simulink model "case14"  (R2018b)
settings: Solver=VariableStepAuto  StartTime=0.0  StopTime=10.0  RelTol=1e-3
(part 1 of 2)
settings Model: Creator=yogita.g  LastModifiedBy=nishanthkumar.l
settings DataIOCC: SaveCompleteFinalSimState=on

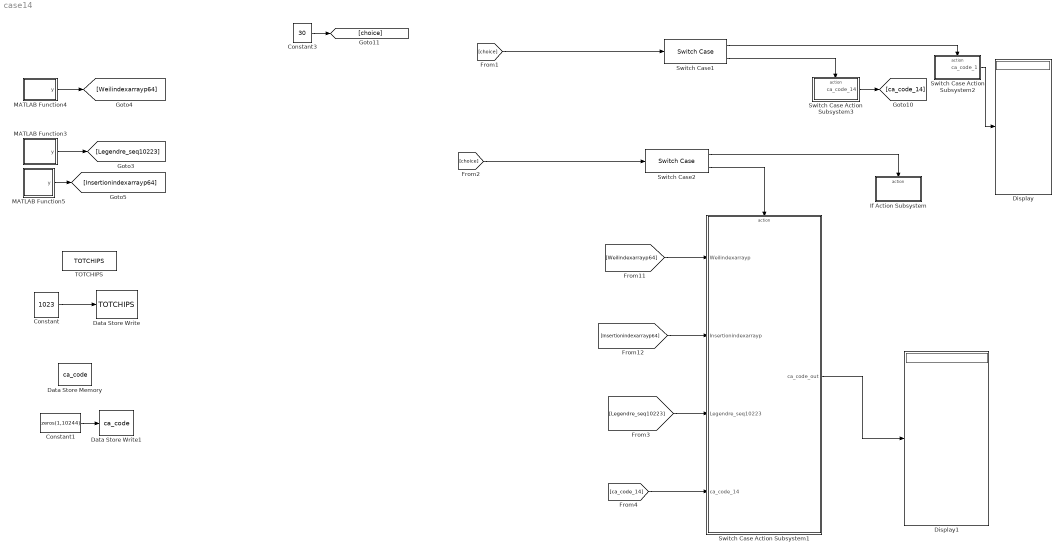
== system case14 ==
  Constant : Constant  Value=1023  VectorParams1D=off  OutDataTypeStr=int32  SampleTime=-1
  Constant1 : Constant  Value=zeros(1,10244)
  Constant3 : Constant  Value=30
  Data Store Memory : DataStoreMemory  DataStoreName=ca_code  ReadBeforeWriteMsg=warning  WriteAfterWriteMsg=warning  WriteAfterReadMsg=warning  ShowAdditionalParam=off  Dimensions=[1 10244]
  Data Store Write : DataStoreWrite  DataStoreName=TOTCHIPS
  Data Store Write1 : DataStoreWrite  DataStoreName=ca_code
  Display : Display
  Display1 : Display
  If Action Subsystem : Subsystem  TreatAsAtomicUnit=on
  MATLAB Function3 : MATLAB Function  TreatAsAtomicUnit=on
  MATLAB Function4 : MATLAB Function  TreatAsAtomicUnit=on
  MATLAB Function5 : MATLAB Function  TreatAsAtomicUnit=on
  Switch Case Action Subsystem1 : Subsystem  TreatAsAtomicUnit=on
  Switch Case Action Subsystem2 : Subsystem  TreatAsAtomicUnit=on
  Switch Case Action Subsystem3 : Subsystem  TreatAsAtomicUnit=on
  Switch Case1 : SwitchCase  CaseConditions={1,14}  ShowDefaultCase=off
  Switch Case2 : SwitchCase  CaseConditions={1,14}  ShowDefaultCase=off
  TOTCHIPS : DataStoreMemory  DataStoreName=TOTCHIPS  ReadBeforeWriteMsg=warning  WriteAfterWriteMsg=warning  WriteAfterReadMsg=warning  ShowAdditionalParam=off  OutDataTypeStr=int32
  wires:
  MATLAB Function5/1(y) -> [Insertionindexarrayp64]
  MATLAB Function4/1(y) -> [Weilindexarrayp64]
  MATLAB Function3/1(y) -> [Legendre_seq10223]
  Switch Case1/1 -> Switch Case Action Subsystem2/Action
  Switch Case1/2 -> Switch Case Action Subsystem3/Action
  Switch Case Action Subsystem3/1(ca_code_14) -> [ca_code_14]
  [choice] -> Switch Case1/1
  Constant3/1 -> [choice]
  Constant/1 -> Data Store Write/1
  Switch Case Action Subsystem2/1(ca_code_1) -> Display/1
  [Weilindexarrayp64] -> Switch Case Action Subsystem1/1(Weilindexarrayp)
  [ca_code_14] -> Switch Case Action Subsystem1/4(ca_code_14)
  [Legendre_seq10223] -> Switch Case Action Subsystem1/3(Legendre_seq10223)
  [Insertionindexarrayp64] -> Switch Case Action Subsystem1/2(Insertionindexarrayp)
  [choice] -> Switch Case2/1
  Switch Case2/2 -> Switch Case Action Subsystem1/Action
  Switch Case2/1 -> If Action Subsystem/Action
  Switch Case Action Subsystem1/1(ca_code_out) -> Display1/1
  Constant1/1 -> Data Store Write1/1

== system case14/If Action Subsystem ==
  Action Port : ActionPort  ActionType=case

== system case14/Switch Case Action Subsystem1 ==
  Weilindexarrayp : Inport
  Insertionindexarrayp : Inport  Port=2
  Legendre_seq10223 : Inport  Port=3
  ca_code_14 : Inport  Port=4
  Action Port : ActionPort  ActionType=case
  For Iterator Subsystem : Subsystem  TreatAsAtomicUnit=on
  ca_code_out : Outport
  wires:
  Weilindexarrayp/1 -> For Iterator Subsystem/1(Weilindexarrayp)
  Insertionindexarrayp/1 -> For Iterator Subsystem/2(Insertionindexarrayp)
  For Iterator Subsystem/1(ca_code) -> ca_code_out/1
  Legendre_seq10223/1 -> For Iterator Subsystem/3(Legendre_seq10223)
  ca_code_14/1 -> For Iterator Subsystem/4(ca_code_14)

== system case14/Switch Case Action Subsystem2 ==
  Action Port : ActionPort  ActionType=case
  MATLAB Function : MATLAB Function  TreatAsAtomicUnit=on
  ca_code_1 : Outport
  wires:
  MATLAB Function/1(ca_code) -> ca_code_1/1

== system case14/Switch Case Action Subsystem3 ==
  Action Port : ActionPort  ActionType=case
  MATLAB Function : MATLAB Function  TreatAsAtomicUnit=on
  ca_code_14 : Outport
  wires:
  MATLAB Function/1(ca_code) -> ca_code_14/1

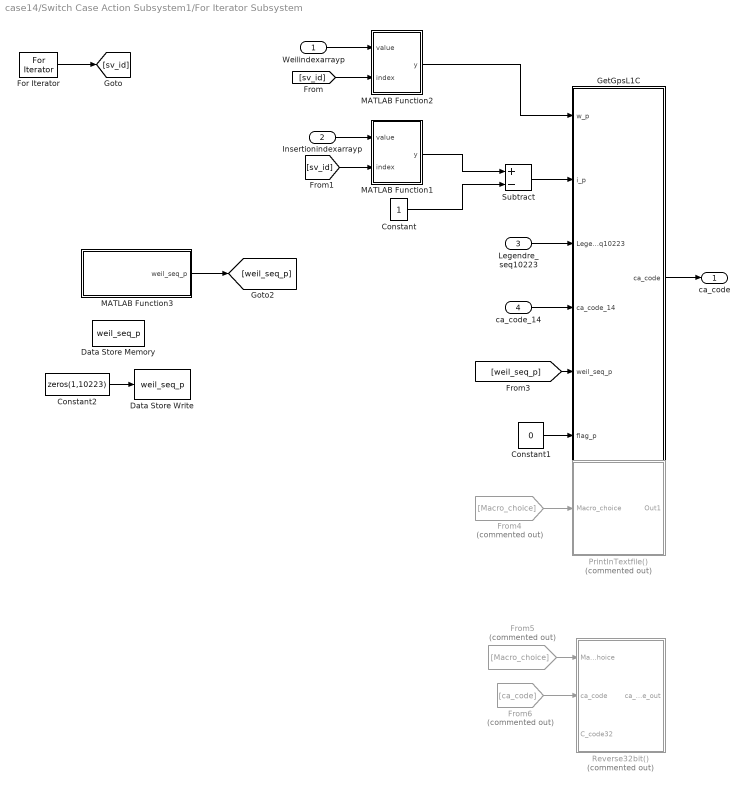
== system case14/Switch Case Action Subsystem1/For Iterator Subsystem ==
  Weilindexarrayp : Inport
  Insertionindexarrayp : Inport  Port=2  OutDataTypeStr=int32
  Legendre_seq10223 : Inport  Port=3
  ca_code_14 : Inport  Port=4
  Constant : Constant  VectorParams1D=off  OutDataTypeStr=int32  SampleTime=-1
  Constant1 : Constant  Value=0  OutDataTypeStr=int32
  Constant2 : Constant  Value=zeros(1,10223)
  Data Store Memory : DataStoreMemory  DataStoreName=weil_seq_p  ReadBeforeWriteMsg=warning  WriteAfterWriteMsg=warning  WriteAfterReadMsg=warning  ShowAdditionalParam=off  Dimensions=[1 10223]
  Data Store Write : DataStoreWrite  DataStoreName=weil_seq_p
  For Iterator : ForIterator  IterationLimit=1
  From4 : From  Commented=on  GotoTag=Macro_choice
  From5 : From  Commented=on  GotoTag=Macro_choice
  From6 : From  Commented=on  GotoTag=ca_code
  GetGpsL1C : Subsystem
  MATLAB Function1 : MATLAB Function  TreatAsAtomicUnit=on
  MATLAB Function2 : MATLAB Function  TreatAsAtomicUnit=on
  MATLAB Function3 : MATLAB Function  TreatAsAtomicUnit=on
  PrintInTextfile() : Subsystem  Commented=on
  Reverse32bit() : Subsystem  Commented=on
  Subtract : Sum  Inputs=+-
  ca_code : Outport
  wires:
  For Iterator/1 -> [sv_id]
  Weilindexarrayp/1 -> MATLAB Function2/1(value)
  [sv_id] -> MATLAB Function2/2(index)
  MATLAB Function2/1(y) -> GetGpsL1C/1(w_p)
  [sv_id] -> MATLAB Function1/2(index)
  Insertionindexarrayp/1 -> MATLAB Function1/1(value)
  From6/1 -> Reverse32bit()/2(ca_code)
  From5/1 -> Reverse32bit()/1(Macro_choice)
  From4/1 -> PrintInTextfile()/1(Macro_choice)
  Legendre_seq10223/1 -> GetGpsL1C/3(Legendre_seq10223)
  GetGpsL1C/1(ca_code) -> ca_code/1
  ca_code_14/1 -> GetGpsL1C/4(ca_code_14)
  [weil_seq_p] -> GetGpsL1C/5(weil_seq_p)
  MATLAB Function1/1(y) -> Subtract/1
  Constant/1 -> Subtract/2
  Subtract/1 -> GetGpsL1C/2(i_p)
  MATLAB Function3/1(weil_seq_p) -> [weil_seq_p]
  Constant1/1 -> GetGpsL1C/6(flag_p)
  Constant2/1 -> Data Store Write/1

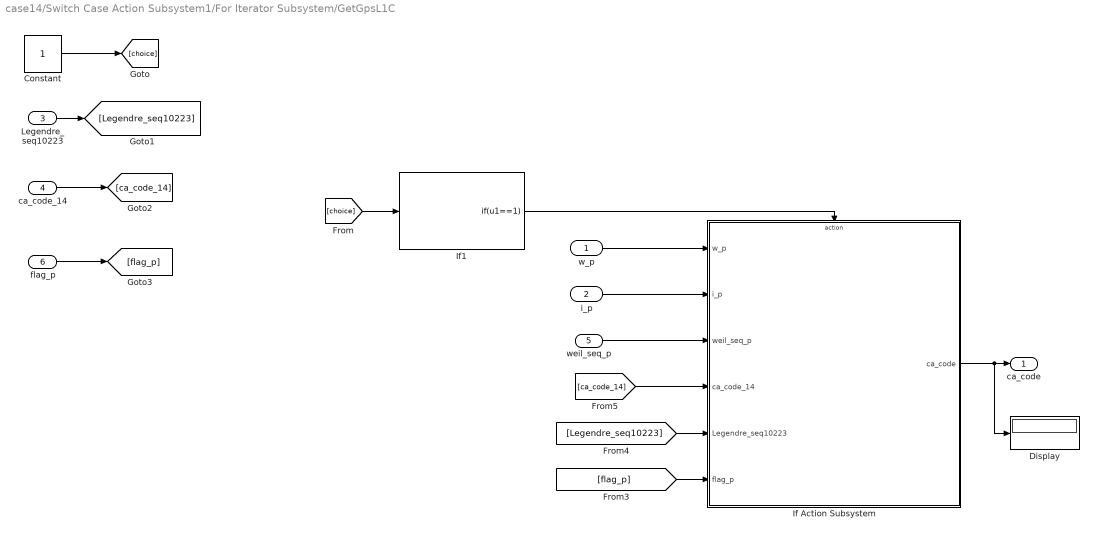
== system case14/Switch Case Action Subsystem1/For Iterator Subsystem/GetGpsL1C ==
  w_p : Inport
  i_p : Inport  Port=2
  Legendre_seq10223 : Inport  Port=3
  ca_code_14 : Inport  Port=4
  weil_seq_p : Inport  Port=5
  flag_p : Inport  Port=6  OutDataTypeStr=int32
  Constant : Constant  VectorParams1D=off  SampleTime=-1
  Display : Display
  If Action Subsystem : Subsystem  TreatAsAtomicUnit=on
  If1 : If  IfExpression=u1==1  ShowElse=off
  ca_code : Outport
  wires:
  If1/1 -> If Action Subsystem/Action
  i_p/1 -> If Action Subsystem/2(i_p)
  [Legendre_seq10223] -> If Action Subsystem/5(Legendre_seq10223)
  w_p/1 -> If Action Subsystem/1(w_p)
  [choice] -> If1/1
  Constant/1 -> [choice]
  Legendre_seq10223/1 -> [Legendre_seq10223]
  If Action Subsystem/1(ca_code) -> Display/1, ca_code/1
  ca_code_14/1 -> [ca_code_14]
  [ca_code_14] -> If Action Subsystem/4(ca_code_14)
  weil_seq_p/1 -> If Action Subsystem/3(weil_seq_p)
  flag_p/1 -> [flag_p]
  [flag_p] -> If Action Subsystem/6(flag_p)

== system case14/Switch Case Action Subsystem1/For Iterator Subsystem/PrintInTextfile() ==
  Macro_choice : Inport
  For Iterator Subsystem : Subsystem  TreatAsAtomicUnit=on
  Out1 : Outport
  wires:
  Macro_choice/1 -> For Iterator Subsystem/1(Macro_choice)

== system case14/Switch Case Action Subsystem1/For Iterator Subsystem/Reverse32bit() ==
  Macro_choice : Inport
  ca_code : Inport  Port=2
  C_code32 : Inport  Port=3
  ConvertChar2hex : Subsystem
  For Iterator Subsystem : Subsystem  TreatAsAtomicUnit=on
  ca_code_out : Outport
  wires:
  Macro_choice/1 -> For Iterator Subsystem/1(Macro_choice)
  ca_code/1 -> For Iterator Subsystem/2(ca_code)
  For Iterator Subsystem/1(ca_code_out) -> ca_code_out/1
  C_code32/1 -> ConvertChar2hex/1(C_code32)

== system case14/Switch Case Action Subsystem1/For Iterator Subsystem/GetGpsL1C/If Action Subsystem ==
  w_p : Inport
  i_p : Inport  Port=2
  weil_seq_p : Inport  Port=3
  ca_code_14 : Inport  Port=4
  Legendre_seq10223 : Inport  Port=5
  flag_p : Inport  Port=6
  Action Port : ActionPort  ActionType=then
  Subsystem : Subsystem
  ca_code : Outport
  wires:
  w_p/1 -> Subsystem/1(w_p)
  i_p/1 -> Subsystem/2(i_p)
  Legendre_seq10223/1 -> Subsystem/4(Legendre_seq10223)
  Subsystem/1(ca_code[]) -> ca_code/1
  ca_code_14/1 -> Subsystem/3(ca_code_14)
  weil_seq_p/1 -> Subsystem/5(weil_seq_p)
  flag_p/1 -> Subsystem/6(flag_p)

== system case14/Switch Case Action Subsystem1/For Iterator Subsystem/PrintInTextfile()/For Iterator Subsystem ==
  Macro_choice : Inport
  For Iterator : ForIterator  ExternalIncrement=on
  Out1 : Outport
  wires:
  Macro_choice/1 -> For Iterator/1

== system case14/Switch Case Action Subsystem1/For Iterator Subsystem/Reverse32bit()/ConvertChar2hex ==
  C_code32 : Inport
  For Iterator Subsystem : Subsystem  TreatAsAtomicUnit=on
  WriteInDatfile : Subsystem
  wires:
  C_code32/1 -> For Iterator Subsystem/1(C_code32)

== system case14/Switch Case Action Subsystem1/For Iterator Subsystem/Reverse32bit()/For Iterator Subsystem ==
  Macro_choice : Inport
  ca_code : Inport  Port=2
  For Iterator : ForIterator  ExternalIncrement=on
  For Iterator Subsystem : Subsystem  TreatAsAtomicUnit=on
  ca_code_out : Outport
  wires:
  Macro_choice/1 -> For Iterator/1
  For Iterator/1 -> For Iterator Subsystem/1(index)
  ca_code/1 -> For Iterator Subsystem/2(ca_code)
  For Iterator Subsystem/1(ca_code_out) -> ca_code_out/1

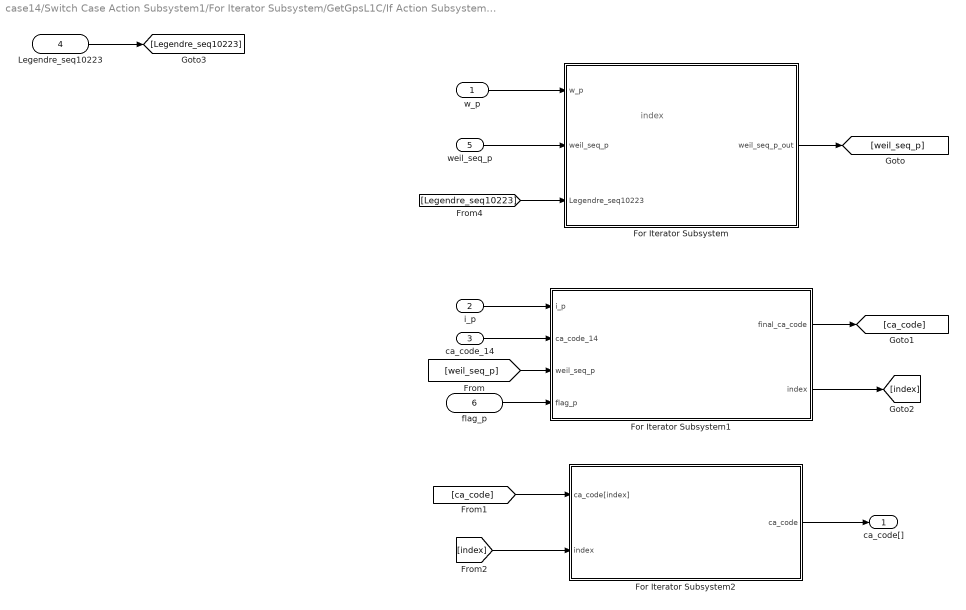
== system case14/Switch Case Action Subsystem1/For Iterator Subsystem/GetGpsL1C/If Action Subsystem/Subsystem ==
  note: index
  w_p : Inport
  i_p : Inport  Port=2
  ca_code_14 : Inport  Port=3
  Legendre_seq10223 : Inport  Port=4
  weil_seq_p : Inport  Port=5
  flag_p : Inport  Port=6
  For Iterator Subsystem : Subsystem  TreatAsAtomicUnit=on
  For Iterator Subsystem1 : Subsystem  TreatAsAtomicUnit=on
  For Iterator Subsystem2 : Subsystem  TreatAsAtomicUnit=on
  ca_code[] : Outport
  wires:
  w_p/1 -> For Iterator Subsystem/1(w_p)
  For Iterator Subsystem/1(weil_seq_p_out) -> [weil_seq_p]
  i_p/1 -> For Iterator Subsystem1/1(i_p)
  For Iterator Subsystem1/1(final_ca_code) -> [ca_code]
  [ca_code] -> For Iterator Subsystem2/1(ca_code[index])
  For Iterator Subsystem2/1(ca_code) -> ca_code[]/1
  For Iterator Subsystem1/2(index) -> [index]
  [index] -> For Iterator Subsystem2/2("index ")
  Legendre_seq10223/1 -> [Legendre_seq10223]
  [Legendre_seq10223] -> For Iterator Subsystem/3(Legendre_seq10223)
  ca_code_14/1 -> For Iterator Subsystem1/2(ca_code_14)
  weil_seq_p/1 -> For Iterator Subsystem/2(weil_seq_p)
  [weil_seq_p] -> For Iterator Subsystem1/3(weil_seq_p)
  flag_p/1 -> For Iterator Subsystem1/4(flag_p)

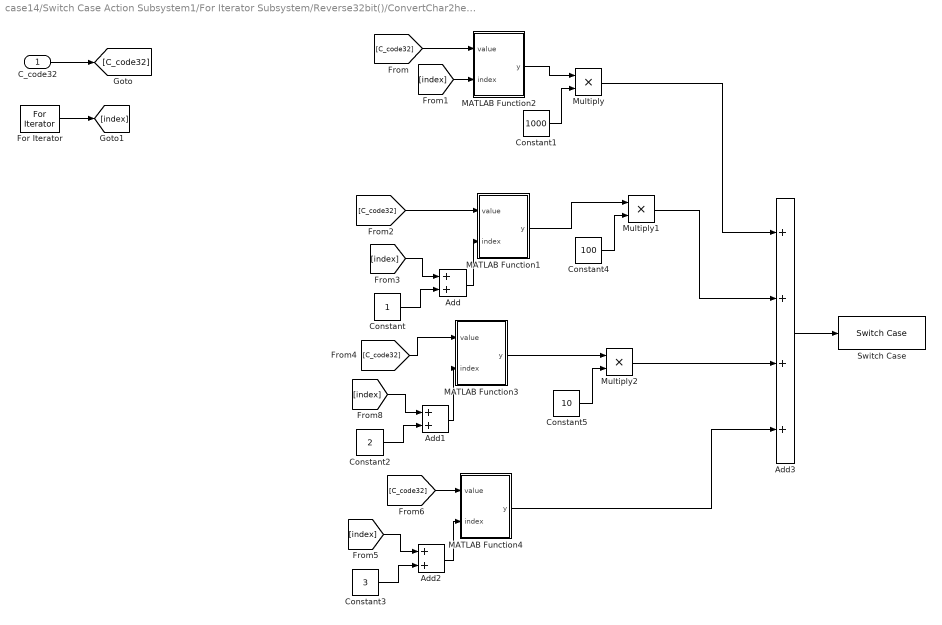
== system case14/Switch Case Action Subsystem1/For Iterator Subsystem/Reverse32bit()/ConvertChar2hex/For Iterator Subsystem ==
  C_code32 : Inport
  Add : Sum
  Add1 : Sum
  Add2 : Sum
  Add3 : Sum  Inputs=++++
  Constant : Constant
  Constant1 : Constant  Value=1000
  Constant2 : Constant  Value=2
  Constant3 : Constant  Value=3
  Constant4 : Constant  Value=100
  Constant5 : Constant  Value=10
  For Iterator : ForIterator  IterationLimit=29
  MATLAB Function1 : MATLAB Function  TreatAsAtomicUnit=on
  MATLAB Function2 : MATLAB Function  TreatAsAtomicUnit=on
  MATLAB Function3 : MATLAB Function  TreatAsAtomicUnit=on
  MATLAB Function4 : MATLAB Function  TreatAsAtomicUnit=on
  Multiply : Product
  Multiply1 : Product
  Multiply2 : Product
  Switch Case : SwitchCase
  wires:
  C_code32/1 -> [C_code32]
  [C_code32] -> MATLAB Function2/1(value)
  For Iterator/1 -> [index]
  [index] -> MATLAB Function2/2(index)
  [C_code32] -> MATLAB Function1/1(value)
  [C_code32] -> MATLAB Function3/1(value)
  [C_code32] -> MATLAB Function4/1(value)
  [index] -> Add/1
  Constant/1 -> Add/2
  Add/1 -> MATLAB Function1/2(index)
  MATLAB Function2/1(y) -> Multiply/1
  Constant1/1 -> Multiply/2
  Constant2/1 -> Add1/2
  [index] -> Add1/1
  Add1/1 -> MATLAB Function3/2(index)
  [index] -> Add2/1
  Constant3/1 -> Add2/2
  Add2/1 -> MATLAB Function4/2(index)
  Constant4/1 -> Multiply1/2
  Constant5/1 -> Multiply2/2
  MATLAB Function3/1(y) -> Multiply2/1
  MATLAB Function1/1(y) -> Multiply1/1
  MATLAB Function4/1(y) -> Add3/4
  Multiply2/1 -> Add3/3
  Multiply1/1 -> Add3/2
  Multiply/1 -> Add3/1
  Add3/1 -> Switch Case/1

== system case14/Switch Case Action Subsystem1/For Iterator Subsystem/Reverse32bit()/ConvertChar2hex/WriteInDatfile ==
  In1 : Inport
  Out1 : Outport
  wires:
  In1/1 -> Out1/1

== system case14/Switch Case Action Subsystem1/For Iterator Subsystem/Reverse32bit()/For Iterator Subsystem/For Iterator Subsystem ==
  index : Inport
  ca_code : Inport  Port=2
  Add : Sum
  Constant : Constant  Value=31
  For Iterator : ForIterator  ExternalIncrement=on
  MATLAB Function : MATLAB Function  TreatAsAtomicUnit=on
  MATLAB Function1 : MATLAB Function  TreatAsAtomicUnit=on
  MATLAB Function2 : MATLAB Function  TreatAsAtomicUnit=on
  Minus : Sum  Inputs=+-
  ca_code_out : Outport
  wires:
  MATLAB Function/1(y) -> For Iterator/1
  For Iterator/1 -> Add/1, Minus/2
  index/1 -> Add/2
  Add/1 -> MATLAB Function2/2(index)
  ca_code/1 -> MATLAB Function2/1(value)
  Constant/1 -> Minus/1
  MATLAB Function2/1(y) -> MATLAB Function1/1(value)
  Minus/1 -> MATLAB Function1/2(index)
  MATLAB Function1/1(y) -> ca_code_out/1

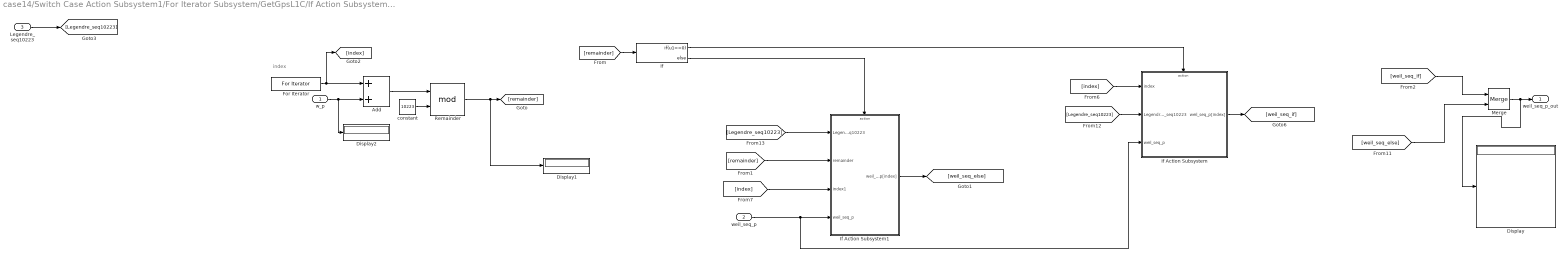
== system case14/Switch Case Action Subsystem1/For Iterator Subsystem/GetGpsL1C/If Action Subsystem/Subsystem/For Iterator Subsystem ==
  note: index
  w_p : Inport
  weil_seq_p : Inport  Port=2
  Legendre_seq10223 : Inport  Port=3
  Add : Sum
  Display : Display
  Display1 : Display
  Display2 : Display
  For Iterator : ForIterator  IterationLimit=10223
  If : If  IfExpression=u1==0
  If Action Subsystem : Subsystem  TreatAsAtomicUnit=on
  If Action Subsystem1 : Subsystem  TreatAsAtomicUnit=on
  Merge : Merge  InitialOutput=[0]
  Remainder : Math  Operator=mod  SaturateOnIntegerOverflow=on
  constant : Constant  Value=10223
  weil_seq_p_out : Outport  InitialOutput=[0]
  wires:
  w_p/1 -> Display2/1, Add/2
  Add/1 -> Remainder/1
  constant/1 -> Remainder/2
  [remainder] -> If/1
  If/1 -> If Action Subsystem/Action
  For Iterator/1 -> [index], Add/1
  Legendre_seq10223/1 -> [Legendre_seq10223]
  [index] -> If Action Subsystem/1(index)
  If/2 -> If Action Subsystem1/Action
  If Action Subsystem/1(weil_seq_p[index]) -> [weil_seq_if]
  [weil_seq_if] -> Merge/1
  Merge/1 -> Display/1, weil_seq_p_out/1
  [Legendre_seq10223] -> If Action Subsystem/2(Legendre_seq10223)
  weil_seq_p/1 -> If Action Subsystem/3(weil_seq_p), If Action Subsystem1/4(weil_seq_p)
  [index] -> If Action Subsystem1/3(index1)
  If Action Subsystem1/1(weil_seq_p[index]) -> [weil_seq_else]
  Remainder/1 -> Display1/1, [remainder]
  [remainder] -> If Action Subsystem1/2(remainder)
  [Legendre_seq10223] -> If Action Subsystem1/1(Legendre_seq10223)
  [weil_seq_else] -> Merge/2

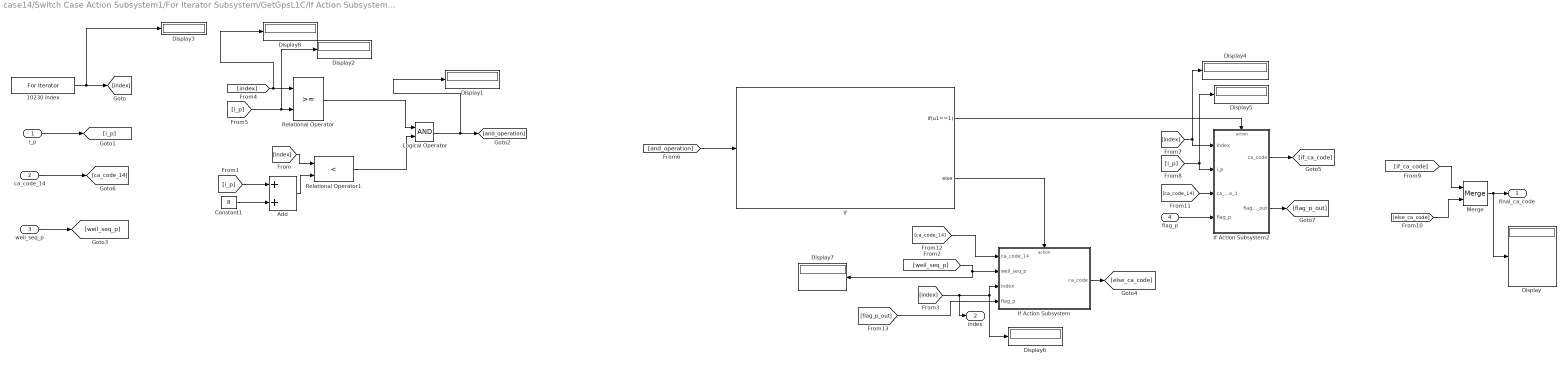
== system case14/Switch Case Action Subsystem1/For Iterator Subsystem/GetGpsL1C/If Action Subsystem/Subsystem/For Iterator Subsystem1 ==
  i_p : Inport  OutDataTypeStr=int32
  ca_code_14 : Inport  Port=2
  weil_seq_p : Inport  Port=3
  flag_p : Inport  Port=4  OutDataTypeStr=int32
  10230 index : ForIterator  IterationLimit=10230
  Add : Sum
  Constant1 : Constant  Value=8  OutDataTypeStr=int32
  Display{,1..8} (9 alike) : Display
  If : If  IfExpression=u1==1
  If Action Subsystem : Subsystem  TreatAsAtomicUnit=on
  If Action Subsystem2 : Subsystem  TreatAsAtomicUnit=on
  Logical Operator : Logic  AllPortsSameDT=off  OutDataTypeStr=boolean
  Merge : Merge
  Relational Operator : RelationalOperator  OutDataTypeStr=boolean  RndMeth=Nearest
  Relational Operator1 : RelationalOperator  Operator=<  OutDataTypeStr=boolean  RndMeth=Nearest
  final_ca_code : Outport
  index : Outport  Port=2
  wires:
  Constant1/1 -> Add/2
  10230 index/1 -> Display3/1, [index]
  Relational Operator/1 -> Logical Operator/1
  Relational Operator1/1 -> Logical Operator/2
  Add/1 -> Relational Operator1/2
  [index] -> Relational Operator1/1
  [i_p] -> Add/1
  If/2 -> If Action Subsystem/Action
  i_p/1 -> [i_p]
  [index] -> Display8/1, Relational Operator/1
  [i_p] -> Display2/1, Relational Operator/2
  Logical Operator/1 -> Display1/1, [and_operation]
  [and_operation] -> If/1
  [index] -> Display4/1, If Action Subsystem2/1(index)
  [i_p] -> If Action Subsystem2/2(i_p), Display5/1
  If/1 -> If Action Subsystem2/Action
  [weil_seq_p] -> Display7/1, If Action Subsystem/2(weil_seq_p)
  [index] -> index/1, Display6/1, If Action Subsystem/3(index)
  If Action Subsystem/1(ca_code) -> [else_ca_code]
  If Action Subsystem2/1("ca_code ") -> [if_ca_code]
  Merge/1 -> final_ca_code/1, Display/1
  [if_ca_code] -> Merge/1
  [else_ca_code] -> Merge/2
  ca_code_14/1 -> [ca_code_14]
  [ca_code_14] -> If Action Subsystem2/3(ca_code_1)
  [ca_code_14] -> If Action Subsystem/1(ca_code_14)
  weil_seq_p/1 -> [weil_seq_p]
  If Action Subsystem2/2("flag_p_out ") -> [flag_p_out]
  [flag_p_out] -> If Action Subsystem/4(flag_p)
  flag_p/1 -> If Action Subsystem2/4(flag_p)

== system case14/Switch Case Action Subsystem1/For Iterator Subsystem/GetGpsL1C/If Action Subsystem/Subsystem/For Iterator Subsystem2 ==
  ca_code[index] : Inport
  "index " : Inport  Port=2
  Display{,1..3} (4 alike) : Display
  For Iterator : ForIterator  IterationLimit=10
  MATLAB Function : MATLAB Function  TreatAsAtomicUnit=on
  ca_code : Outport
  wires:
  For Iterator/1 -> [index1]
  ca_code[index]/1 -> [ca_code]
  "index "/1 -> [index]
  [ca_code] -> Display3/1, MATLAB Function/1("value ")
  MATLAB Function/1(value) -> Display2/1, ca_code/1
  [index1] -> MATLAB Function/3(index1), Display1/1
  [index] -> Display/1, MATLAB Function/2(index)

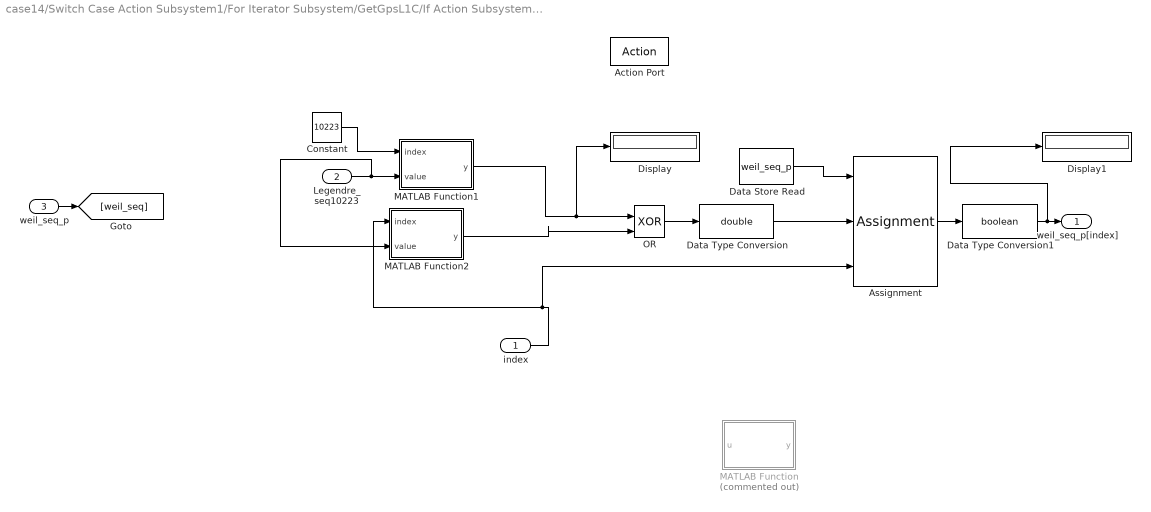
== system case14/Switch Case Action Subsystem1/For Iterator Subsystem/GetGpsL1C/If Action Subsystem/Subsystem/For Iterator Subsystem/If Action Subsystem ==
  index : Inport
  Legendre_seq10223 : Inport  Port=2
  weil_seq_p : Inport  Port=3
  Action Port : ActionPort  ActionType=then
  Assignment : Assignment  DiagnosticForDimensions=Warning  IndexOptions=Index vector (port)  Indices=[1:1023]  OutputSizes=1
  Constant : Constant  Value=10223
  Data Store Read : DataStoreRead  DataStoreName=weil_seq_p
  Data Type Conversion : DataTypeConversion  OutDataTypeStr=double
  Data Type Conversion1 : DataTypeConversion  OutDataTypeStr=boolean
  Display : Display
  Display1 : Display
  MATLAB Function : MATLAB Function  Commented=on  TreatAsAtomicUnit=on
  MATLAB Function1 : MATLAB Function  TreatAsAtomicUnit=on
  MATLAB Function2 : MATLAB Function  TreatAsAtomicUnit=on
  OR : Logic  Operator=XOR  IconShape=distinctive  AllPortsSameDT=off  OutDataTypeStr=boolean
  weil_seq_p[index] : Outport
  wires:
  MATLAB Function2/1(y) -> OR/2
  Constant/1 -> MATLAB Function1/1(index)
  Legendre_seq10223/1 -> MATLAB Function2/2(value), MATLAB Function1/2(value)
  MATLAB Function1/1(y) -> Display/1, OR/1
  Data Store Read/1 -> Assignment/1
  index/1 -> Assignment/3, MATLAB Function2/1(index)
  weil_seq_p/1 -> [weil_seq]
  OR/1 -> Data Type Conversion/1
  Data Type Conversion/1 -> Assignment/2
  Assignment/1 -> Data Type Conversion1/1
  Data Type Conversion1/1 -> Display1/1, weil_seq_p[index]/1

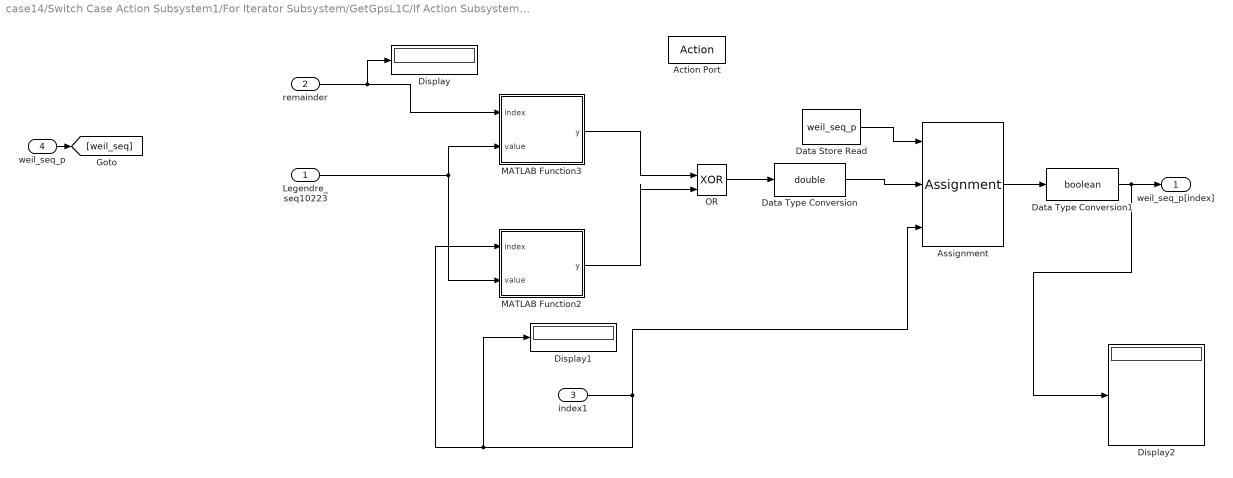
== system case14/Switch Case Action Subsystem1/For Iterator Subsystem/GetGpsL1C/If Action Subsystem/Subsystem/For Iterator Subsystem/If Action Subsystem1 ==
  Legendre_seq10223 : Inport
  remainder : Inport  Port=2
  index1 : Inport  Port=3
  weil_seq_p : Inport  Port=4
  Action Port : ActionPort  ActionType=else
  Assignment : Assignment  DiagnosticForDimensions=Warning  IndexOptions=Index vector (port)  Indices=[1:1023]  OutputSizes=1
  Data Store Read : DataStoreRead  DataStoreName=weil_seq_p
  Data Type Conversion : DataTypeConversion  OutDataTypeStr=double
  Data Type Conversion1 : DataTypeConversion  OutDataTypeStr=boolean
  Display : Display
  Display1 : Display
  Display2 : Display
  MATLAB Function2 : MATLAB Function  TreatAsAtomicUnit=on
  MATLAB Function3 : MATLAB Function  TreatAsAtomicUnit=on
  OR : Logic  Operator=XOR  IconShape=distinctive  AllPortsSameDT=off  OutDataTypeStr=boolean
  weil_seq_p[index] : Outport
  wires:
  index1/1 -> MATLAB Function2/1(index), Display1/1, Assignment/3
  Legendre_seq10223/1 -> MATLAB Function3/2(value), MATLAB Function2/2(value)
  MATLAB Function3/1(y) -> OR/1
  MATLAB Function2/1(y) -> OR/2
  remainder/1 -> Display/1, MATLAB Function3/1(index)
  OR/1 -> Data Type Conversion/1
  Data Type Conversion/1 -> Assignment/2
  Data Store Read/1 -> Assignment/1
  weil_seq_p/1 -> [weil_seq]
  Assignment/1 -> Data Type Conversion1/1
  Data Type Conversion1/1 -> Display2/1, weil_seq_p[index]/1

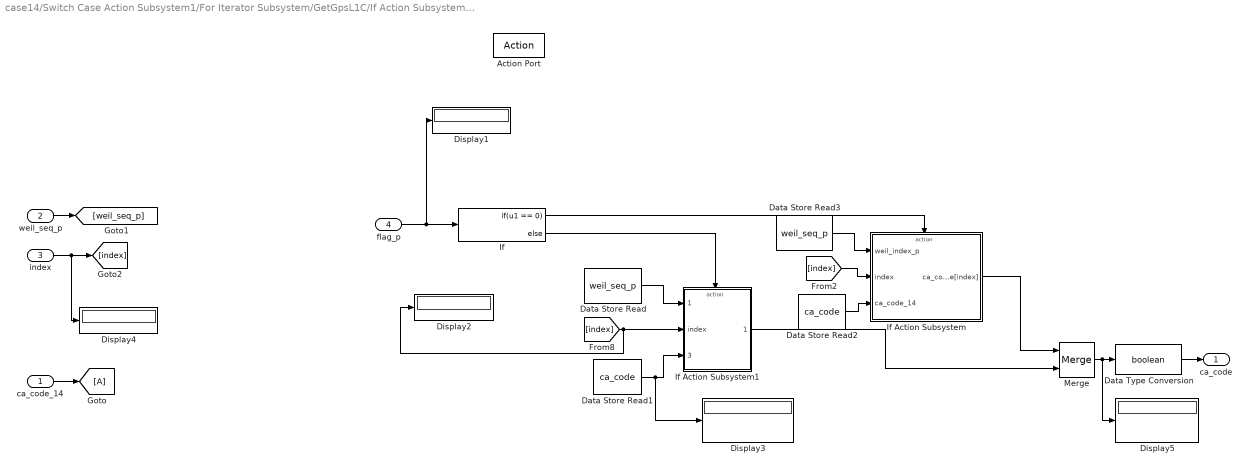
== system case14/Switch Case Action Subsystem1/For Iterator Subsystem/GetGpsL1C/If Action Subsystem/Subsystem/For Iterator Subsystem1/If Action Subsystem ==
  ca_code_14 : Inport
  weil_seq_p : Inport  Port=2
  index : Inport  Port=3
  flag_p : Inport  Port=4
  Action Port : ActionPort  ActionType=else
  Data Store Read : DataStoreRead  DataStoreName=weil_seq_p
  Data Store Read1 : DataStoreRead  DataStoreName=ca_code
  Data Store Read2 : DataStoreRead  DataStoreName=ca_code
  Data Store Read3 : DataStoreRead  DataStoreName=weil_seq_p
  Data Type Conversion : DataTypeConversion  OutDataTypeStr=boolean
  Display{1..5} (5 alike) : Display
  If : If  IfExpression=u1 == 0
  If Action Subsystem : Subsystem  TreatAsAtomicUnit=on
  If Action Subsystem1 : Subsystem  TreatAsAtomicUnit=on
  Merge : Merge
  ca_code : Outport
  wires:
  flag_p/1 -> Display1/1, If/1
  If/1 -> If Action Subsystem/Action
  If/2 -> If Action Subsystem1/Action
  weil_seq_p/1 -> [weil_seq_p]
  index/1 -> Display4/1, [index]
  [index] -> If Action Subsystem/2(index)
  Merge/1 -> Display5/1, Data Type Conversion/1
  If Action Subsystem/1(ca_code[index]) -> Merge/1
  If Action Subsystem1/1(ca_code) -> Merge/2
  Data Store Read/1 -> If Action Subsystem1/1(weil_seq_p)
  [index] -> Display2/1, If Action Subsystem1/2(index)
  ca_code_14/1 -> [A]
  Data Store Read1/1 -> Display3/1, If Action Subsystem1/3(ca_code_14)
  Data Store Read2/1 -> If Action Subsystem/3(ca_code_14)
  Data Store Read3/1 -> If Action Subsystem/1(weil_index_p)
  Data Type Conversion/1 -> ca_code/1

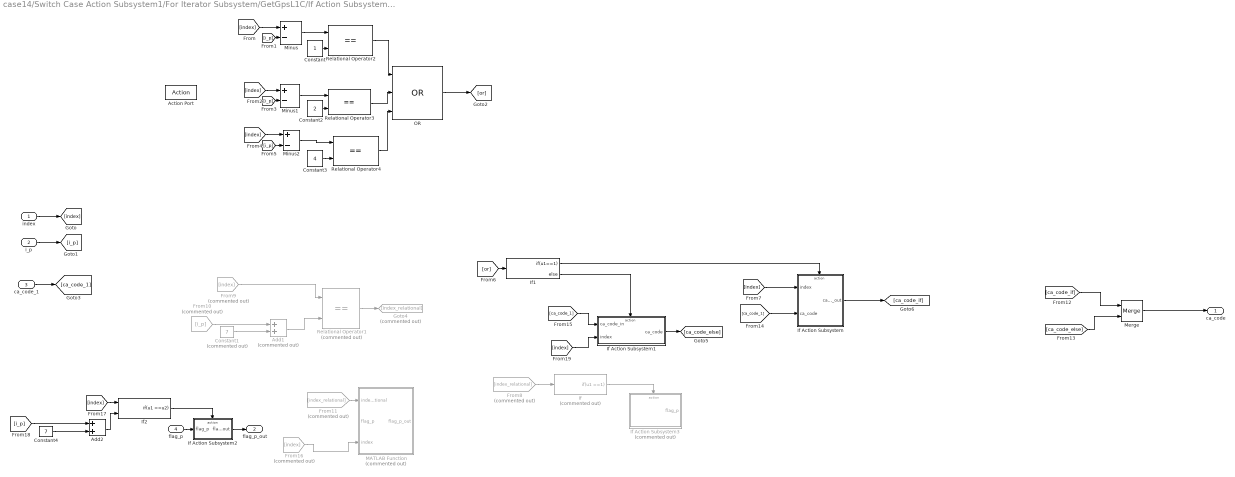
== system case14/Switch Case Action Subsystem1/For Iterator Subsystem/GetGpsL1C/If Action Subsystem/Subsystem/For Iterator Subsystem1/If Action Subsystem2 ==
  index : Inport
  i_p : Inport  Port=2  OutDataTypeStr=int32
  ca_code_1 : Inport  Port=3
  flag_p : Inport  Port=4  OutDataTypeStr=int32
  Action Port : ActionPort  ActionType=then
  Add1 : Sum  Commented=on
  Add2 : Sum
  Constant : Constant
  Constant1 : Constant  Commented=on  Value=7
  Constant2 : Constant  Value=2
  Constant3 : Constant  Value=4
  Constant4 : Constant  Value=7  OutDataTypeStr=int32
  From10 : From  Commented=on  GotoTag=i_p
  From11 : From  Commented=on  GotoTag=index_relational
  From16 : From  Commented=on  GotoTag=index
  From8 : From  Commented=on  GotoTag=index_relational
  From9 : From  Commented=on  GotoTag=index
  Goto4 : Goto  Commented=on  GotoTag=index_relational
  If : If  Commented=on  IfExpression=u1 ==1  ShowElse=off
  If Action Subsystem : Subsystem  TreatAsAtomicUnit=on
  If Action Subsystem1 : Subsystem  TreatAsAtomicUnit=on
  If Action Subsystem2 : Subsystem  TreatAsAtomicUnit=on
  If Action Subsystem3 : Subsystem  Commented=on  TreatAsAtomicUnit=on
  If1 : If  IfExpression=u1==1
  If2 : If  NumInputs=2  IfExpression=u1 ==u2  ShowElse=off
  MATLAB Function : MATLAB Function  Commented=on  TreatAsAtomicUnit=on
  Merge : Merge
  Minus : Sum  Inputs=+-
  Minus1 : Sum  Inputs=+-
  Minus2 : Sum  Inputs=+-
  OR : Logic  Operator=OR  Inputs=3  IconShape=distinctive  AllPortsSameDT=off  OutDataTypeStr=boolean
  Relational Operator1 : RelationalOperator  Commented=on  Operator===  OutDataTypeStr=boolean  RndMeth=Nearest
  Relational Operator2 : RelationalOperator  Operator===  OutDataTypeStr=boolean  RndMeth=Nearest
  Relational Operator3 : RelationalOperator  Operator===  OutDataTypeStr=boolean  RndMeth=Nearest
  Relational Operator4 : RelationalOperator  Operator===  OutDataTypeStr=boolean  RndMeth=Nearest
  "ca_code " : Outport
  "flag_p_out " : Outport  Port=2  OutDataTypeStr=int32
  wires:
  If1/2 -> If Action Subsystem1/Action
  [i_p] -> Minus1/2
  [i_p] -> Minus/2
  Constant/1 -> Relational Operator2/2
  Constant3/1 -> Relational Operator4/2
  Relational Operator4/1 -> OR/3
  Relational Operator3/1 -> OR/2
  [i_p] -> Minus2/2
  Minus1/1 -> Relational Operator3/1
  [index] -> Minus1/1
  Constant2/1 -> Relational Operator3/2
  Relational Operator2/1 -> OR/1
  [index] -> Minus2/1
  Minus/1 -> Relational Operator2/1
  Minus2/1 -> Relational Operator4/1
  [index] -> Minus/1
  index/1 -> [index]
  i_p/1 -> [i_p]
  OR/1 -> [or]
  [or] -> If1/1
  If1/1 -> If Action Subsystem/Action
  [index] -> If Action Subsystem/1("index ")
  From10/1 -> Add1/1
  Constant1/1 -> Add1/2
  Add1/1 -> Relational Operator1/2
  From9/1 -> Relational Operator1/1
  Relational Operator1/1 -> Goto4/1
  If Action Subsystem1/1(ca_code) -> [ca_code_else]
  If Action Subsystem/1(ca_code_out) -> [ca_code_if]
  [ca_code_if] -> Merge/1
  [ca_code_else] -> Merge/2
  Merge/1 -> "ca_code "/1
  ca_code_1/1 -> [ca_code_1]
  [ca_code_1] -> If Action Subsystem/2(ca_code)
  [ca_code_1] -> If Action Subsystem1/1(ca_code_in)
  If/1 -> If Action Subsystem3/Action
  From8/1 -> If/1
  From11/1 -> MATLAB Function/1(index_relational)
  From16/1 -> MATLAB Function/3(index)
  [index] -> If2/1
  Constant4/1 -> Add2/2
  [i_p] -> Add2/1
  Add2/1 -> If2/2
  flag_p/1 -> If Action Subsystem2/1(flag_p)
  If2/1 -> If Action Subsystem2/Action
  If Action Subsystem2/1("flag_p_out ") -> "flag_p_out "/1
  [index] -> If Action Subsystem1/2(index)

== system case14/Switch Case Action Subsystem1/For Iterator Subsystem/GetGpsL1C/If Action Subsystem/Subsystem/For Iterator Subsystem1/If Action Subsystem/If Action Subsystem ==
  weil_index_p : Inport
  index : Inport  Port=2
  ca_code_14 : Inport  Port=3
  Action Port : ActionPort  ActionType=then
  Assignment : Assignment  DiagnosticForDimensions=Warning  IndexOptions=Index vector (port)  Indices=[1:1023]  OutputSizes=1
  Data Store Read : DataStoreRead  DataStoreName=ca_code
  Data Store Read1 : DataStoreRead  DataStoreName=weil_seq_p
  Display : Display
  MATLAB Function : MATLAB Function  Commented=on  TreatAsAtomicUnit=on
  MATLAB Function1 : MATLAB Function  TreatAsAtomicUnit=on
  ca_code[index] : Outport
  wires:
  Data Store Read/1 -> Assignment/1
  Data Store Read1/1 -> MATLAB Function1/1(value)
  index/1 -> Assignment/3, MATLAB Function1/2(index)
  MATLAB Function1/1(y) -> Assignment/2
  Assignment/1 -> Display/1, ca_code[index]/1
  weil_index_p/1 -> [A1]
  ca_code_14/1 -> [A]

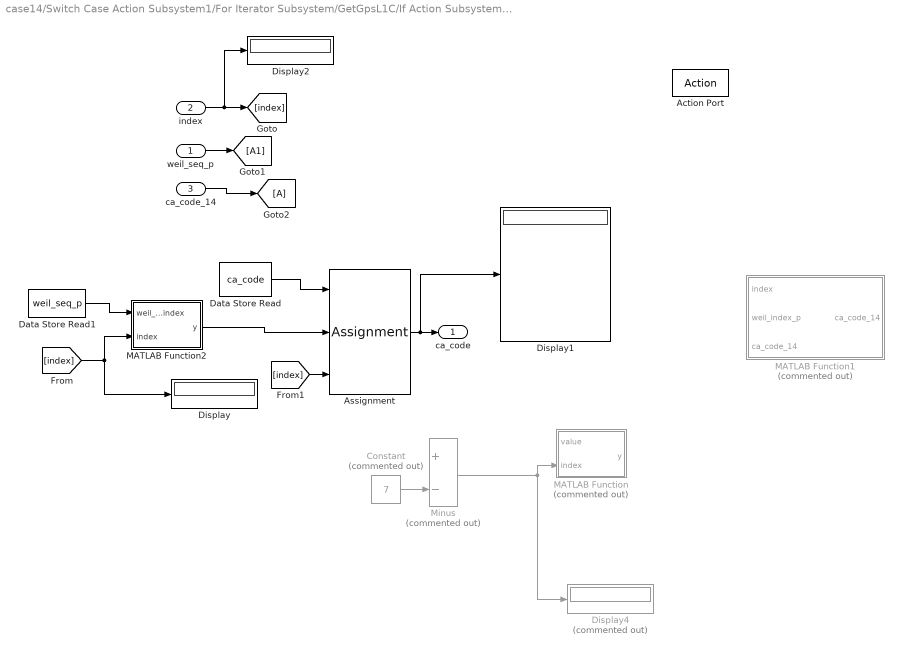
== system case14/Switch Case Action Subsystem1/For Iterator Subsystem/GetGpsL1C/If Action Subsystem/Subsystem/For Iterator Subsystem1/If Action Subsystem/If Action Subsystem1 ==
  weil_seq_p : Inport
  index : Inport  Port=2
  ca_code_14 : Inport  Port=3
  Action Port : ActionPort  ActionType=else
  Assignment : Assignment  DiagnosticForDimensions=Warning  IndexOptions=Index vector (port)  Indices=[1:1023]  OutputSizes=1
  Constant : Constant  Commented=on  Value=7
  Data Store Read : DataStoreRead  DataStoreName=ca_code
  Data Store Read1 : DataStoreRead  DataStoreName=weil_seq_p
  Display : Display
  Display1 : Display
  Display2 : Display
  Display4 : Display  Commented=on
  MATLAB Function : MATLAB Function  Commented=on  TreatAsAtomicUnit=on
  MATLAB Function1 : MATLAB Function  Commented=on  TreatAsAtomicUnit=on
  MATLAB Function2 : MATLAB Function  TreatAsAtomicUnit=on
  Minus : Sum  Commented=on  Inputs=+-
  ca_code : Outport
  wires:
  index/1 -> Display2/1, [index]
  Constant/1 -> Minus/2
  Minus/1 -> Display4/1, MATLAB Function/2(index)
  [index] -> MATLAB Function2/2(index), Display/1
  Data Store Read/1 -> Assignment/1
  MATLAB Function2/1(y) -> Assignment/2
  Data Store Read1/1 -> MATLAB Function2/1(weil_seq_p_index)
  [index] -> Assignment/3
  Assignment/1 -> Display1/1, ca_code/1
  weil_seq_p/1 -> [A1]
  ca_code_14/1 -> [A]

== system case14/Switch Case Action Subsystem1/For Iterator Subsystem/GetGpsL1C/If Action Subsystem/Subsystem/For Iterator Subsystem1/If Action Subsystem2/If Action Subsystem ==
  "index " : Inport
  ca_code : Inport  Port=2
  Action Port : ActionPort  ActionType=then
  Assignment : Assignment  Commented=on  DiagnosticForDimensions=Warning  IndexOptions=Index vector (port)  Indices=[1:1023]  OutputSizes=1
  Assignment1 : Assignment  DiagnosticForDimensions=Warning  IndexOptions=Index vector (port)  Indices=[1:1023]  OutputSizes=1
  Constant : Constant
  Data Store Read : DataStoreRead  DataStoreName=ca_code
  Data Type Conversion : DataTypeConversion  Commented=on  OutDataTypeStr=double
  Data Type Conversion1 : DataTypeConversion  OutDataTypeStr=boolean
  Display : Display
  MATLAB Function : MATLAB Function  Commented=on  TreatAsAtomicUnit=on
  MATLAB Function15 : MATLAB Function  Commented=on  TreatAsAtomicUnit=on
  ca_code_out : Outport
  wires:
  MATLAB Function15/1(ca_code) -> Assignment/1
  Data Type Conversion/1 -> Assignment/2
  Data Store Read/1 -> Assignment1/1
  "index "/1 -> Assignment1/3
  Constant/1 -> Assignment1/2
  ca_code/1 -> [A]
  Assignment1/1 -> Data Type Conversion1/1
  Data Type Conversion1/1 -> Display/1, ca_code_out/1

== system case14/Switch Case Action Subsystem1/For Iterator Subsystem/GetGpsL1C/If Action Subsystem/Subsystem/For Iterator Subsystem1/If Action Subsystem2/If Action Subsystem1 ==
  ca_code_in : Inport
  index : Inport  Port=2
  Action Port : ActionPort  ActionType=else
  Assignment : Assignment  DiagnosticForDimensions=Warning  IndexOptions=Index vector (port)  Indices=[1:1023]  OutputSizes=1
  Constant : Constant  Value=0
  Data Store Read : DataStoreRead  DataStoreName=ca_code
  Data Type Conversion : DataTypeConversion  OutDataTypeStr=boolean
  Display : Display
  ca_code : Outport
  wires:
  Data Store Read/1 -> Assignment/1
  Constant/1 -> Assignment/2
  index/1 -> Assignment/3
  ca_code_in/1 -> [A]
  Assignment/1 -> Data Type Conversion/1
  Data Type Conversion/1 -> Display/1, ca_code/1

== system case14/Switch Case Action Subsystem1/For Iterator Subsystem/GetGpsL1C/If Action Subsystem/Subsystem/For Iterator Subsystem1/If Action Subsystem2/If Action Subsystem2 ==
  flag_p : Inport
  Action Port : ActionPort  ActionType=then
  Display : Display
  MATLAB Function : MATLAB Function  TreatAsAtomicUnit=on
  "flag_p_out " : Outport  OutDataTypeStr=int32
  wires:
  flag_p/1 -> MATLAB Function/1(u)
  MATLAB Function/1(y) -> Display/1, "flag_p_out "/1

== system case14/Switch Case Action Subsystem1/For Iterator Subsystem/GetGpsL1C/If Action Subsystem/Subsystem/For Iterator Subsystem1/If Action Subsystem2/If Action Subsystem3 ==
  Action Port : ActionPort
  Constant : Constant  Commented=on
  Constant1 : Constant
  Data Store Write : DataStoreWrite  Commented=on  DataStoreName=Flag_p
  flag_p : Outport
  wires:
  Constant/1 -> Data Store Write/1
  Constant1/1 -> flag_p/1

== matlab function case14/Switch Case Action Subsystem1/For Iterator Subsystem/GetGpsL1C/If Action Subsystem/Subsystem/For Iterator Subsystem1/If Action Subsystem2/If Action Subsystem/MATLAB Function15 ==
  data: ca_code output
function ca_code = fcn()
ca_code=zeros(1,1023);

== matlab function case14/Switch Case Action Subsystem1/For Iterator Subsystem/GetGpsL1C/If Action Subsystem/Subsystem/For Iterator Subsystem/If Action Subsystem/MATLAB Function ==
  data: u input; y output
function y = fcn(u)
persistent u
y = u;
end
